simulink model "bpsk_rx_time_sync"  (R2019a)
settings: Solver=VariableStepAuto  StartTime=0.0  StopTime=4000/3.2e6  RelTol=1e-3
InitFcn:
  | setup_bpsk_receiver
undefined symbols (not defined in the file): AXI4, designMultirateFIR, Lite, tx_data, xlfda_numerator
libraries: xbsIndex_r4 x34, dspmlti4 x11, hdlsllib x11, dspswit3 x4, dspsigops x2, commrandsrc3 x1, simulink x1
(part 1 of 2)
settings Model: Creator=david  LastModifiedBy=david

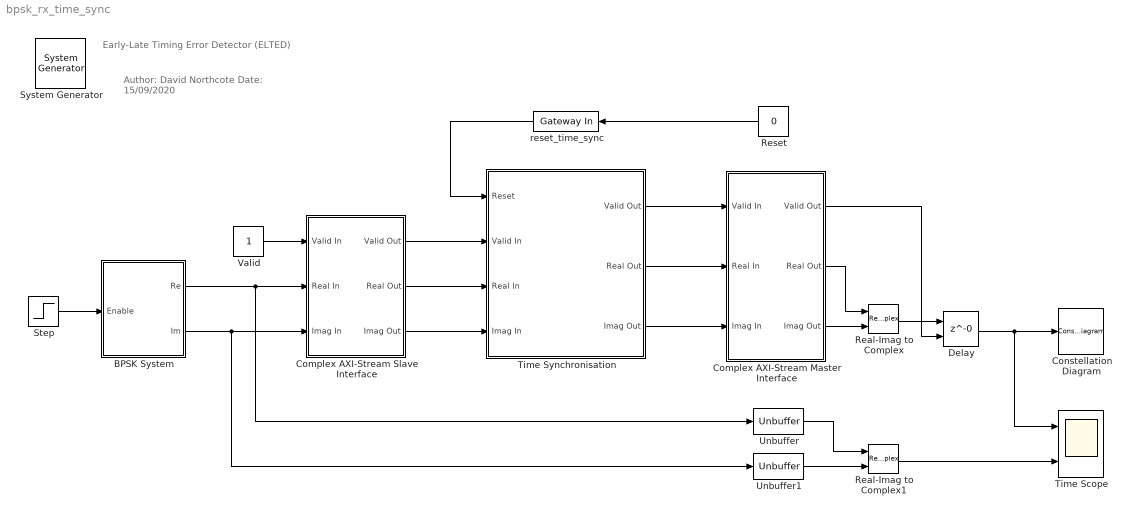
== system bpsk_rx_time_sync ==
  note: Author: 	David Northcote
      | Date: 	15/09/2020
  note: Early-Late Timing Error Detector (ELTED)
  " System Generator" : xbsIndex_r4/ System Generator  Tag=genX  xilinxfamily=zynquplusRFSOC  part=xczu28dr  speed=-2-e  package=ffvg1517  synthesis_tool=Vivado  clock_wrapper=Clock Enables  directory=./netlist  proj_type=Vivado  Synth_file=Vivado Synthesis Defaults  Impl_file=Vivado Implementation Defaults  testbench=off  simulink_period=1/3.2e6  sysclk_period=(1/3.2e6)*1e9  dcm_input_clock_period=10  incr_netlist=off  trim_vbits=Everywhere in SubSystem  dbl_ovrd=According to Block Masks  core_generation=According to Block Masks  run_coregen=off  deprecated_control=off  eval_field=0  block_type=sysgen
  BPSK System : Subsystem
  Complex AXI-Stream Master Interface : Subsystem
  Complex AXI-Stream Slave Interface : Subsystem
  Constellation Diagram : ConstellationDiagram
  Delay : Delay  DelayLength=0  ShowEnablePort=on
      settings: InputPortMap=u0,e6
  Real-Imag to Complex : RealImagToComplex
  Real-Imag to Complex1 : RealImagToComplex
  Reset : Constant  Value=0  OutDataTypeStr=boolean  SampleTime=-1
  Step : Step  Time=4/12.5e3  SampleTime=1/12.5e3
  Time Scope : Scope  NumInputPorts=2
  Time Synchronisation : Subsystem
  Unbuffer : Unbuffer
  Unbuffer1 : Unbuffer
  Valid : Constant  OutDataTypeStr=boolean  SampleTime=1/3.2e6
  reset_time_sync : xbsIndex_r4/Gateway In  gui_display_data_type=Boolean  arith_type=Boolean  n_bits=16  bin_pt=14  preci_type=Single  exp_width=8  frac_width=24  rows=1  columns=1  quantization="Round  (unbiased: +/- Inf)"  overflow=Saturate  period=1/3.2e6  UseAsADC=off  ADCChannel='1'  interface=AXI4-Lite  automatic_assignment=off  address_offset=0  intf_name=''  intf_description=''  default_value=0  timing_constraint=None  locs_specified=off  LOCs={}  io_standard={}  inherit_from_input=off  hdl_port=on  dbl_ovrd=off  block_type=gatewayin
  wires:
  BPSK System/1(Re) -> Unbuffer/1, Complex AXI-Stream Slave Interface/2(Real In)
  BPSK System/2(Im) -> Unbuffer1/1, Complex AXI-Stream Slave Interface/3(Imag In)
  Step/1 -> BPSK System/1(Enable)
  Unbuffer1/1 -> Real-Imag to Complex1/2
  Unbuffer/1 -> Real-Imag to Complex1/1
  Real-Imag to Complex1/1 -> Time Scope/2
  Time Synchronisation/1(Valid Out) -> Complex AXI-Stream Master Interface/1(Valid In)
  Time Synchronisation/2(Real Out) -> Complex AXI-Stream Master Interface/2(Real In)
  Time Synchronisation/3(Imag Out) -> Complex AXI-Stream Master Interface/3(Imag In)
  Complex AXI-Stream Master Interface/2(Real Out) -> Real-Imag to Complex/1
  Complex AXI-Stream Master Interface/3(Imag Out) -> Real-Imag to Complex/2
  Valid/1 -> Complex AXI-Stream Slave Interface/1(Valid In)
  Complex AXI-Stream Slave Interface/1(Valid Out) -> Time Synchronisation/2(Valid In)
  Complex AXI-Stream Slave Interface/2(Real Out) -> Time Synchronisation/3(Real In)
  Complex AXI-Stream Slave Interface/3(Imag Out) -> Time Synchronisation/4(Imag In)
  reset_time_sync/1 -> Time Synchronisation/1(Reset)
  Reset/1 -> reset_time_sync/1
  Real-Imag to Complex/1 -> Delay/1
  Complex AXI-Stream Master Interface/1(Valid Out) -> Delay/2
  Delay/1 -> Constellation Diagram/1, Time Scope/1

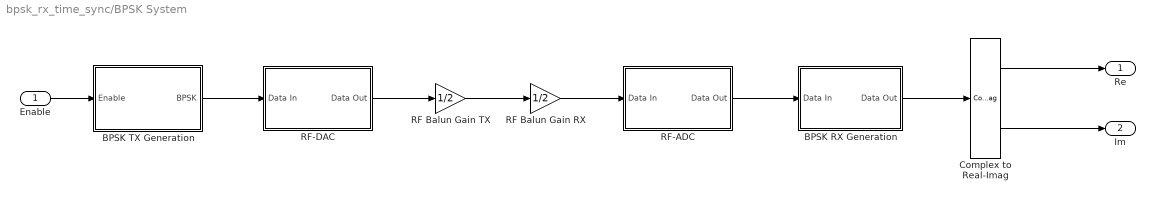
== system bpsk_rx_time_sync/BPSK System ==
  Enable : Inport
  BPSK RX Generation : Subsystem
  BPSK TX Generation : Subsystem
  Complex to Real-Imag : ComplexToRealImag
  RF Balun Gain RX : Gain  Gain=1/2
  RF Balun Gain TX : Gain  Gain=1/2
  RF-ADC : Subsystem  mask{fs_ghz=1.024, decim=8x, ssr=2, mode=Fine, fc=0.064, fph=0, fcoarse=fs/4}
      mask prompts: fs_ghz "Sample Rate (GHz):"; decim "Interpolation Mode:"; ssr "Samples per AXI4-Stream Cycle:"; mode "Mixer Type:"; fc "NCO Frequency (GHz):"; fph "NCO Phase (Rads):"; fcoarse "Frequency:"
      mask init:
      | % Obtain the sample rate in Hz
      | fs = str2double(get_param(gcb, 'fs_ghz'))*1e9;
      | 
      | % Set the mode of the RF-DAC interpolation filter
      | switch get_param(gcb, 'decim')
      |     case '1x'
      |         D = 1;
      |     case '2x'
      |         D = 2;
      |     case '4x'
      |         D = 4;
      |     case '8x'
      |         D = 8;
      |     otherwise
      |         D = 1;
      | end
      | 
      | % Get the AXI-Stream clock for display to user
      | axi_clk = (fs/(str2double(get_param(gcb, 'ssr'))*D))*1e-6;
      | 
      | % Get the block mask object to manipulate settings
      | mo = get_param(gcb, 'MaskObject');
      | 
      | % Update text to display the required AXI-Stream clock
      | tc = mo.getDialogControl('axi_text');
      | tc.Prompt = ['      Required AXI-Stream Clock: ', num2str(axi_clk), ' MHz'];
      | 
      | % Set the RF-DAC Mixer mode
      | switch get_param(gcb, 'mode')
      |     case 'Bypass'
      |         m = 0;
      |     case 'Coarse'
      |         m = 1;
      |     case 'Fine'
      |         m = 2;
      |     otherwise
      |         m = 0;
      | end
      | 
      | % Set the RF-DAC Coarse Mixer mode
      | switch get_param(gcb, 'fcoarse')
      |     case 'fs/2'
      |         mc = 0;
      |     case 'fs/4'
      |         mc = 1;
      |     case '-fs/4'
      |         mc = 2;
      |     otherwise
      |         mc = 0;
      | end
      | 
      | % Set other blocks
      | set_param([gcb, '/Decimation Filter'], 'decim', get_param(gcb, 'decim'));
      mask Callback fs_ghz:
      | % Obtain the sample rate in Hz
      | fs = str2double(get_param(gcb, 'fs_ghz'))*1e9;
      | 
      | % Set the mode of the RF-DAC interpolation filter
      | switch get_param(gcb, 'decim')
      |     case '1x'
      |         D = 1;
      |     case '2x'
      |         D = 2;
      |     case '4x'
      |         D = 4;
      |     case '8x'
      |         D = 8;
      |     otherwise
      |         D = 1;
      | end
      | 
      | % Get the AXI-Stream clock for display to user
      | axi_clk = (fs/(str2double(get_param(gcb, 'ssr'))*D))*1e-6;
      | 
      | % Get the block mask object to manipulate settings
      | mo = get_param(gcb, 'MaskObject');
      | 
      | % Update text to display the required AXI-Stream clock
      | tc = mo.getDialogControl('axi_text');
      | tc.Prompt = ['      Required AXI-Stream Clock: ', num2str(axi_clk), ' MHz'];
      mask TypeOptions decim: 1x | 2x | 4x | 8x
      mask Callback decim:
      | % Obtain the sample rate in Hz
      | fs = str2double(get_param(gcb, 'fs_ghz'))*1e9;
      | 
      | % Set the mode of the RF-DAC interpolation filter
      | switch get_param(gcb, 'decim')
      |     case '1x'
      |         D = 1;
      |     case '2x'
      |         D = 2;
      |     case '4x'
      |         D = 4;
      |     case '8x'
      |         D = 8;
      |     otherwise
      |         D = 1;
      | end
      | 
      | % Get the AXI-Stream clock for display to user
      | axi_clk = (fs/(str2double(get_param(gcb, 'ssr'))*D))*1e-6;
      | 
      | % Get the block mask object to manipulate settings
      | mo = get_param(gcb, 'MaskObject');
      | 
      | % Update text to display the required AXI-Stream clock
      | tc = mo.getDialogControl('axi_text');
      | tc.Prompt = ['      Required AXI-Stream Clock: ', num2str(axi_clk), ' MHz'];
      mask TypeOptions ssr: 1 | 2 | 3 | 4 | 5 | 6 | 7 | 8 | 9 | 10 | 11 | 12 | 13 | 14 | 15 | 16
      mask Callback ssr:
      | % Obtain the sample rate in Hz
      | fs = str2double(get_param(gcb, 'fs_ghz'))*1e9;
      | 
      | % Set the mode of the RF-DAC interpolation filter
      | switch get_param(gcb, 'decim')
      |     case '1x'
      |         D = 1;
      |     case '2x'
      |         D = 2;
      |     case '4x'
      |         D = 4;
      |     case '8x'
      |         D = 8;
      |     otherwise
      |         D = 1;
      | end
      | 
      | % Get the AXI-Stream clock for display to user
      | axi_clk = (fs/(str2double(get_param(gcb, 'ssr'))*D))*1e-6;
      | 
      | % Get the block mask object to manipulate settings
      | mo = get_param(gcb, 'MaskObject');
      | 
      | % Update text to display the required AXI-Stream clock
      | tc = mo.getDialogControl('axi_text');
      | tc.Prompt = ['      Required AXI-Stream Clock: ', num2str(axi_clk), ' MHz'];
      mask TypeOptions mode: Coarse | Fine
      mask Callback mode:
      | % Get the block mask object to manipulate settings
      | mo = get_param(gcb, 'MaskObject');
      | 
      | % Hide group depending on Mixer mode choice
      | switch get_param(gcb, 'mode')
      |     case 'Bypass'
      |         mo.getDialogControl('coarse_group').Visible='off';
      |         mo.getDialogControl('mixer_group').Visible='off';
      |     case 'Coarse'
      |         mo.getDialogControl('coarse_group').Visible='on';
      |         mo.getDialogControl('mixer_group').Visible='off';
      |     case 'Fine'
      |         mo.getDialogControl('coarse_group').Visible='off';
      |         mo.getDialogControl('mixer_group').Visible='on';
      |     otherwise
      |         mo.getDialogControl('coarse_group').Visible='off';
      |         mo.getDialogControl('mixer_group').Visible='off';
      | end
      mask TypeOptions fcoarse: fs/2 | fs/4 | -fs/4
      mask DialogControl DescGroupVar Prompt: RF-DAC
      mask DialogControl DescTextVar Prompt: This block simulates one RF-ADC channel.
      mask DialogControl main_group Prompt: Data Settings
      mask DialogControl axi_text Prompt: Required AXI-Stream Clock: 64 MHz
      mask DialogControl Container5 Prompt: Mixer Settings
  RF-DAC : Subsystem  mask{fs_ghz=1.024, interp=8x, ssr=1, mode=Fine, fc=0.064, fph=0, fcoarse=fs/4}
      mask prompts: fs_ghz "Sample Rate (GHz):"; interp "Interpolation Mode:"; ssr "Samples per AXI4-Stream Cycle:"; mode "Mixer Type:"; fc "NCO Frequency (GHz):"; fph "NCO Phase (Rads):"; fcoarse "Frequency:"
      mask init:
      | % Obtain the sample rate in Hz
      | fs = str2double(get_param(gcb, 'fs_ghz'))*1e9;
      | 
      | % Set the mode of the RF-DAC interpolation filter
      | switch get_param(gcb, 'interp')
      |     case '1x'
      |         L = 1;
      |     case '2x'
      |         L = 2;
      |     case '4x'
      |         L = 4;
      |     case '8x'
      |         L = 8;
      |     otherwise
      |         L = 1;
      | end
      | 
      | % Get the AXI-Stream clock for display to user
      | axi_clk = (fs/(str2double(get_param(gcb, 'ssr'))*L))*1e-6;
      | 
      | % Get the block mask object to manipulate settings
      | mo = get_param(gcb, 'MaskObject');
      | 
      | % Update text to display the required AXI-Stream clock
      | tc = mo.getDialogControl('axi_text');
      | tc.Prompt = ['      Required AXI-Stream Clock: ', num2str(axi_clk), ' MHz'];
      | 
      | % Set the RF-DAC Mixer mode
      | switch get_param(gcb, 'mode')
      |     case 'Bypass'
      |         m = 0;
      |     case 'Coarse'
      |         m = 1;
      |     case 'Fine'
      |         m = 2;
      |     otherwise
      |         m = 0;
      | end
      | 
      | % Set the RF-DAC Coarse Mixer mode
      | switch get_param(gcb, 'fcoarse')
      |     case 'fs/2'
      |         mc = 0;
      |     case 'fs/4'
      |         mc = 1;
      |     case '-fs/4'
      |         mc = 2;
      |     otherwise
      |         mc = 0;
      | end
      | 
      | % Set other blocks
      | set_param([gcb, '/Interpolation Filter'], 'interp', get_param(gcb, 'interp'));
      mask Callback fs_ghz:
      | % Obtain the sample rate in Hz
      | fs = str2double(get_param(gcb, 'fs_ghz'))*1e9;
      | 
      | % Set the mode of the RF-DAC interpolation filter
      | switch get_param(gcb, 'interp')
      |     case '1x'
      |         L = 1;
      |     case '2x'
      |         L = 2;
      |     case '4x'
      |         L = 4;
      |     case '8x'
      |         L = 8;
      |     otherwise
      |         L = 1;
      | end
      | 
      | % Get the AXI-Stream clock for display to user
      | axi_clk = (fs/(str2double(get_param(gcb, 'ssr'))*L))*1e-6;
      | 
      | % Get the block mask object to manipulate settings
      | mo = get_param(gcb, 'MaskObject');
      | 
      | % Update text to display the required AXI-Stream clock
      | tc = mo.getDialogControl('axi_text');
      | tc.Prompt = ['      Required AXI-Stream Clock: ', num2str(axi_clk), ' MHz'];
      mask TypeOptions interp: 1x | 2x | 4x | 8x
      mask Callback interp:
      | % Obtain the sample rate in Hz
      | fs = str2double(get_param(gcb, 'fs_ghz'))*1e9;
      | 
      | % Set the mode of the RF-DAC interpolation filter
      | switch get_param(gcb, 'interp')
      |     case '1x'
      |         L = 1;
      |     case '2x'
      |         L = 2;
      |     case '4x'
      |         L = 4;
      |     case '8x'
      |         L = 8;
      |     otherwise
      |         L = 1;
      | end
      | 
      | % Get the AXI-Stream clock for display to user
      | axi_clk = (fs/(str2double(get_param(gcb, 'ssr'))*L))*1e-6;
      | 
      | % Get the block mask object to manipulate settings
      | mo = get_param(gcb, 'MaskObject');
      | 
      | % Update text to display the required AXI-Stream clock
      | tc = mo.getDialogControl('axi_text');
      | tc.Prompt = ['      Required AXI-Stream Clock: ', num2str(axi_clk), ' MHz'];
      mask TypeOptions ssr: 1 | 2 | 3 | 4 | 5 | 6 | 7 | 8 | 9 | 10 | 11 | 12 | 13 | 14 | 15 | 16
      mask Callback ssr:
      | % Obtain the sample rate in Hz
      | fs = str2double(get_param(gcb, 'fs_ghz'))*1e9;
      | 
      | % Set the mode of the RF-DAC interpolation filter
      | switch get_param(gcb, 'interp')
      |     case '1x'
      |         L = 1;
      |     case '2x'
      |         L = 2;
      |     case '4x'
      |         L = 4;
      |     case '8x'
      |         L = 8;
      |     otherwise
      |         L = 1;
      | end
      | 
      | % Get the AXI-Stream clock for display to user
      | axi_clk = (fs/(str2double(get_param(gcb, 'ssr'))*L))*1e-6;
      | 
      | % Get the block mask object to manipulate settings
      | mo = get_param(gcb, 'MaskObject');
      | 
      | % Update text to display the required AXI-Stream clock
      | tc = mo.getDialogControl('axi_text');
      | tc.Prompt = ['      Required AXI-Stream Clock: ', num2str(axi_clk), ' MHz'];
      mask TypeOptions mode: Coarse | Fine
      mask Callback mode:
      | % Get the block mask object to manipulate settings
      | mo = get_param(gcb, 'MaskObject');
      | 
      | % Hide group depending on Mixer mode choice
      | switch get_param(gcb, 'mode')
      |     case 'Bypass'
      |         mo.getDialogControl('coarse_group').Visible='off';
      |         mo.getDialogControl('mixer_group').Visible='off';
      |     case 'Coarse'
      |         mo.getDialogControl('coarse_group').Visible='on';
      |         mo.getDialogControl('mixer_group').Visible='off';
      |     case 'Fine'
      |         mo.getDialogControl('coarse_group').Visible='off';
      |         mo.getDialogControl('mixer_group').Visible='on';
      |     otherwise
      |         mo.getDialogControl('coarse_group').Visible='off';
      |         mo.getDialogControl('mixer_group').Visible='off';
      | end
      mask TypeOptions fcoarse: fs/2 | fs/4 | -fs/4
      mask DialogControl DescGroupVar Prompt: RF-DAC
      mask DialogControl DescTextVar Prompt: This block simulates one RF-DAC channel.
      mask DialogControl main_group Prompt: Data Settings
      mask DialogControl axi_text Prompt: Required AXI-Stream Clock: 128 MHz
      mask DialogControl Container5 Prompt: Mixer Settings
  Re : Outport
  Im : Outport  Port=2
  wires:
  RF Balun Gain RX/1 -> RF-ADC/1(Data In)
  RF Balun Gain TX/1 -> RF Balun Gain RX/1
  RF-DAC/1(Data Out) -> RF Balun Gain TX/1
  Complex to Real-Imag/2 -> Im/1
  Complex to Real-Imag/1 -> Re/1
  Enable/1 -> BPSK TX Generation/1(Enable)
  BPSK TX Generation/1(BPSK) -> RF-DAC/1(Data In)
  RF-ADC/1(Data Out) -> BPSK RX Generation/1(Data In)
  BPSK RX Generation/1(Data Out) -> Complex to Real-Imag/1

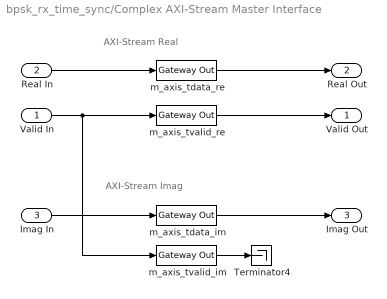
== system bpsk_rx_time_sync/Complex AXI-Stream Master Interface ==
  note: AXI-Stream Real
  note: AXI-Stream Imag
  Valid In : Inport
  Real In : Inport  Port=2
  Imag In : Inport  Port=3
  Terminator4 : Terminator
  m_axis_tdata_im : xbsIndex_r4/Gateway Out  inherit_from_input=off  hdl_port=on  rows=1  columns=1  UseAsDAC=off  DACChannel='1'  interface=None  automatic_assignment=on  address_offset=hex2dec('00')  intf_name=''  intf_description=''  timing_constraint=None  locs_specified=off  LOCs={}  io_standard={}  block_type=gatewayout
  m_axis_tdata_re : xbsIndex_r4/Gateway Out  inherit_from_input=off  hdl_port=on  rows=1  columns=1  UseAsDAC=off  DACChannel='1'  interface=None  automatic_assignment=on  address_offset=hex2dec('00')  intf_name=''  intf_description=''  timing_constraint=None  locs_specified=off  LOCs={}  io_standard={}  block_type=gatewayout
  m_axis_tvalid_im : xbsIndex_r4/Gateway Out  inherit_from_input=off  hdl_port=on  rows=1  columns=1  UseAsDAC=off  DACChannel='1'  interface=None  automatic_assignment=on  address_offset=hex2dec('00')  intf_name=''  intf_description=''  timing_constraint=None  locs_specified=off  LOCs={}  io_standard={}  block_type=gatewayout
  m_axis_tvalid_re : xbsIndex_r4/Gateway Out  inherit_from_input=off  hdl_port=on  rows=1  columns=1  UseAsDAC=off  DACChannel='1'  interface=None  automatic_assignment=on  address_offset=hex2dec('00')  intf_name=''  intf_description=''  timing_constraint=None  locs_specified=off  LOCs={}  io_standard={}  block_type=gatewayout
  Valid Out : Outport
  Real Out : Outport  Port=2
  Imag Out : Outport  Port=3
  wires:
  Real In/1 -> m_axis_tdata_re/1
  m_axis_tdata_im/1 -> Imag Out/1
  m_axis_tvalid_im/1 -> Terminator4/1
  Valid In/1 -> m_axis_tvalid_re/1, m_axis_tvalid_im/1
  m_axis_tdata_re/1 -> Real Out/1
  m_axis_tvalid_re/1 -> Valid Out/1
  Imag In/1 -> m_axis_tdata_im/1

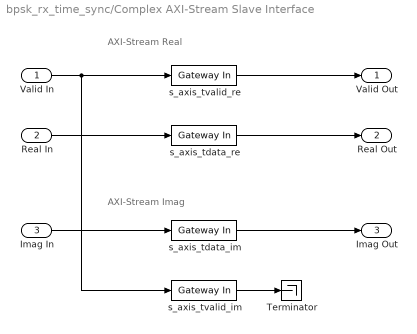
== system bpsk_rx_time_sync/Complex AXI-Stream Slave Interface ==
  note: AXI-Stream Real
  note: AXI-Stream Imag
  Valid In : Inport
  Real In : Inport  Port=2
  Imag In : Inport  Port=3
  Terminator : Terminator
  s_axis_tdata_im : xbsIndex_r4/Gateway In  gui_display_data_type=Fixed-point  arith_type="Signed  (2's comp)"  n_bits=16  bin_pt=14  preci_type=Single  exp_width=8  frac_width=24  rows=1  columns=1  quantization="Round  (unbiased: +/- Inf)"  overflow=Saturate  period=1/3.2e6  UseAsADC=off  ADCChannel='1'  interface=None  automatic_assignment=on  address_offset=hex2dec('00')  intf_name=''  intf_description=''  default_value=0  timing_constraint=None  locs_specified=off  LOCs={}  io_standard={}  inherit_from_input=off  hdl_port=on  dbl_ovrd=off  block_type=gatewayin
  s_axis_tdata_re : xbsIndex_r4/Gateway In  gui_display_data_type=Fixed-point  arith_type="Signed  (2's comp)"  n_bits=16  bin_pt=14  preci_type=Single  exp_width=8  frac_width=24  rows=1  columns=1  quantization="Round  (unbiased: +/- Inf)"  overflow=Saturate  period=1/3.2e6  UseAsADC=off  ADCChannel='1'  interface=None  automatic_assignment=on  address_offset=hex2dec('00')  intf_name=''  intf_description=''  default_value=0  timing_constraint=None  locs_specified=off  LOCs={}  io_standard={}  inherit_from_input=off  hdl_port=on  dbl_ovrd=off  block_type=gatewayin
  s_axis_tvalid_im : xbsIndex_r4/Gateway In  gui_display_data_type=Boolean  arith_type=Boolean  n_bits=16  bin_pt=14  preci_type=Single  exp_width=8  frac_width=24  rows=1  columns=1  quantization="Round  (unbiased: +/- Inf)"  overflow=Saturate  period=1/3.2e6  UseAsADC=off  ADCChannel='1'  interface=None  automatic_assignment=on  address_offset=hex2dec('00')  intf_name=''  intf_description=''  default_value=0  timing_constraint=None  locs_specified=off  LOCs={}  io_standard={}  inherit_from_input=off  hdl_port=on  dbl_ovrd=off  block_type=gatewayin
  s_axis_tvalid_re : xbsIndex_r4/Gateway In  gui_display_data_type=Boolean  arith_type=Boolean  n_bits=16  bin_pt=14  preci_type=Single  exp_width=8  frac_width=24  rows=1  columns=1  quantization="Round  (unbiased: +/- Inf)"  overflow=Saturate  period=1/3.2e6  UseAsADC=off  ADCChannel='1'  interface=None  automatic_assignment=on  address_offset=hex2dec('00')  intf_name=''  intf_description=''  default_value=0  timing_constraint=None  locs_specified=off  LOCs={}  io_standard={}  inherit_from_input=off  hdl_port=on  dbl_ovrd=off  block_type=gatewayin
  Valid Out : Outport
  Real Out : Outport  Port=2
  Imag Out : Outport  Port=3
  wires:
  Imag In/1 -> s_axis_tdata_im/1
  s_axis_tdata_re/1 -> Real Out/1
  s_axis_tdata_im/1 -> Imag Out/1
  Valid In/1 -> s_axis_tvalid_im/1, s_axis_tvalid_re/1
  s_axis_tvalid_re/1 -> Valid Out/1
  s_axis_tvalid_im/1 -> Terminator/1
  Real In/1 -> s_axis_tdata_re/1

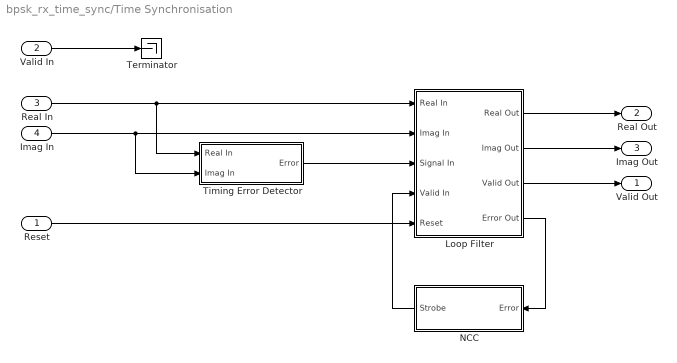
== system bpsk_rx_time_sync/Time Synchronisation ==
  Reset : Inport
  Valid In : Inport  Port=2
  Real In : Inport  Port=3
  Imag In : Inport  Port=4
  Loop Filter : Subsystem  mask{T=1/100e3, d=1/sqrt(2), Kp=3.7, Bn=0.01*100e3, Ko=1}
      mask prompts: T "Sampling Period:"; d "Damping Ratio:"; Kp "Phase Detector Gain:"; Bn "Noise Bandwidth:"; Ko "Oscillator Gain:"
      mask init:
      | n = (Bn*T)/(d+1/(4*d));
      | 
      | K1 = ((4*d*n)/(1+2*d*n+n^2))/(Ko*Kp);
      | 
      | K2 = ((4*n^2)/(1+2*d*n+n^2))/(Ko*Kp);
      | 
      | %K1 = (4*d*n)/(Ko*Kp);
      | 
      | %K2 = (4*(n^2))/(Ko*Kp);
      mask DialogControl DescGroupVar Prompt: Loop Filter
      mask DialogControl DescTextVar Prompt: A simplified loop filter.
      mask DialogControl ParameterGroupVar Prompt: Main
  NCC : Subsystem  mask{r=32}
      mask prompts: r "Symbol Oversample Factor:"
      mask init:
      | n = ceil(log2(r));
      | f = 32-n;
      mask DialogControl DescGroupVar Prompt: Numerically Controlled Clock (NCC)
      mask DialogControl DescTextVar Prompt: The NCC block contains an accumulator that increments by one each clock cycle. The wordlength of the accumulator is determined by the symbol oversampling factor. Once the maximum value of the accumulator is reached, the accumulation starts again. The error signal can be used to increase or decrease the rate of accumulation. When the accumulator wraps around, a binary high is released from the strobe port.
      mask DialogControl ParameterGroupVar Prompt: Main
  Terminator : Terminator
  Timing Error Detector : Subsystem
  Valid Out : Outport
  Real Out : Outport  Port=2
  Imag Out : Outport  Port=3
  wires:
  Reset/1 -> Loop Filter/5(Reset)
  NCC/1(Strobe) -> Loop Filter/4(Valid In)
  Loop Filter/2(Imag Out) -> Imag Out/1
  Loop Filter/1(Real Out) -> Real Out/1
  Loop Filter/3(Valid Out) -> Valid Out/1
  Imag In/1 -> Timing Error Detector/2(Imag In), Loop Filter/2(Imag In)
  Timing Error Detector/1(Error) -> Loop Filter/3(Signal In)
  Loop Filter/4(Error Out) -> NCC/1(Error)
  Real In/1 -> Loop Filter/1(Real In), Timing Error Detector/1(Real In)
  Valid In/1 -> Terminator/1

== system bpsk_rx_time_sync/BPSK System/BPSK RX Generation ==
  Data In : Inport
  CIC Decimation : dspmlti4/CIC Decimation  filtFrom=Dialog parameters  filtobj=CICDECIM  ftype=Decimator  R=5  M=1  N=3  filterInternals=Full precision  BPS=[16 16 16 16]  FLPS=0  outputWordLength=32  outputFracLength=0  launchFVT=off  framing=Maintain input frame rate  RateOptions=Allow multirate processing
      settings: SourceProductName=DSP System Toolbox  SourceProductBaseCode=DS
  FDATool : xbsIndex_r4/FDATool  block_type=fdatool
      settings: infoedit=FDATool
  FIR 0 : dspmlti4/FIR Decimation  FilterSource=Dialog parameters  h=xlfda_numerator('FDATool')/(max(xlfda_numerator('FDATool'))*2)  D=2  filtStruct=Direct form  FilterObject=fir0  framing=Enforce single-rate processing  inputOffset=0  outputBufInitCond=0  roundingMode=Floor  overflowMode=off  firstCoeffDataTypeStr=Inherit: Same word length as input  firstCoeffMin=[]  firstCoeffMax=[]  firstCoeffLastDataTypeStr=Inherit: Same word length as input  outputMode=Binary point scaling  outputWordLength=16  outputFracLength=14  outputDataTypeStr=fixdt(1,16,14)  outputMin=[]  outputMax=[]  outputLastDataTypeStr=fixdt(1,16,14)
  Gain : Gain  Gain=2^(floor(log2(5^3)))/(5^3)  ParamDataTypeStr=fixdt(1,16,14)  OutDataTypeStr=fixdt(1,16,14)
  RRC Receive Filter : Subsystem
  Shift Arithmetic : ArithShift  BitShiftNumber=floor(log2(5^3))  BitShiftDirection=Right
  Unbuffer : Unbuffer
  Data Out : Outport
  wires:
  Unbuffer/1 -> FIR 0/1
  Data In/1 -> Unbuffer/1
  FIR 0/1 -> CIC Decimation/1
  CIC Decimation/1 -> Shift Arithmetic/1
  Shift Arithmetic/1 -> Gain/1
  Gain/1 -> RRC Receive Filter/1(Data In)
  RRC Receive Filter/1(Data Out) -> Data Out/1

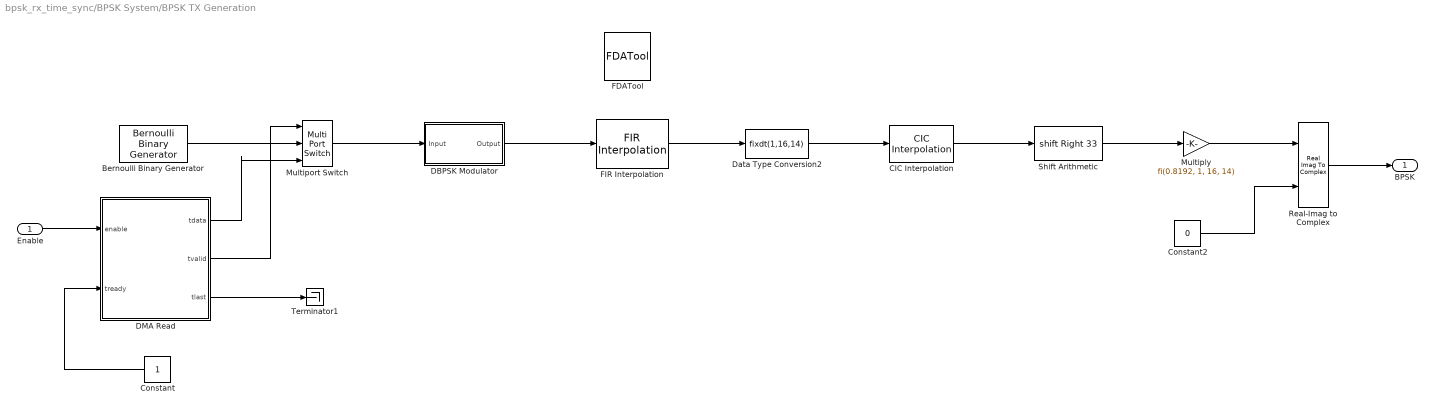
== system bpsk_rx_time_sync/BPSK System/BPSK TX Generation ==
  Enable : Inport
  Bernoulli Binary Generator : commrandsrc3/Bernoulli Binary Generator  ProbabilityOfZero=0.5  SeedSource=Auto  Seed=0  SampleTime=1/100e3  SamplesPerFrame=1  OutputDataType=double  SimulateUsing=Interpreted execution
      settings: SourceProductName=Communications Toolbox
  CIC Interpolation : dspmlti4/CIC Interpolation  filtFrom=Dialog parameters  filtobj=Hm_interp  ftype=Interpolator  R=320  M=1  N=5  filterInternals=Full precision  BPS=[16 16 16 16]  FLPS=0  outputWordLength=32  outputFracLength=0  launchFVT=off  framing=Allow multirate processing  OutputFrames=off
      settings: SourceProductName=DSP System Toolbox  SourceProductBaseCode=DS
  Constant : Constant  SampleTime=1/12.5e3
  Constant2 : Constant  Value=0  OutDataTypeStr=Inherit: Inherit via back propagation  SampleTime=-1
  DBPSK Modulator : Subsystem
  DMA Read : Subsystem
  Data Type Conversion2 : DataTypeConversion  OutDataTypeStr=fixdt(1,16,14)
  FDATool : xbsIndex_r4/FDATool  block_type=fdatool
      settings: infoedit=FDATool
  FIR Interpolation : dspmlti4/FIR Interpolation  FilterSource=Dialog parameters  h=xlfda_numerator('FDATool')/(max(xlfda_numerator('FDATool')))  L=4  FilterObject=xlfda_numerator('FDATool')/(max(xlfda_numerator('FDATool')))  framing=Allow multirate processing  outputBufInitCond=0  roundingMode=Floor  overflowMode=off  firstCoeffMode=Binary point scaling  firstCoeffWordLength=16  firstCoeffFracLength=14  firstCoeffDataTypeStr=fixdt(1,16,14)  firstCoeffMin=[]  firstCoeffMax=[]  firstCoeffLastDataTypeStr=fixdt(1,16,14)  outputDataTypeStr=Inherit: Same as accumulator  outputMin=[]  outputMax=[]  outputLastDataTypeStr=Inherit: Same as accumulator
      settings: SourceProductName=DSP System Toolbox
  Multiply : Gain  Gain=fi(0.8192, 1, 16, 14)  ParamDataTypeStr=fixdt(1,16,15)  OutDataTypeStr=fixdt(1,16,14)
  Multiport Switch : MultiPortSwitch  DataPortOrder=Zero-based contiguous  Inputs=2  zeroidx=on
  Real-Imag to Complex : RealImagToComplex
  Shift Arithmetic : ArithShift  BitShiftNumber=33  BitShiftDirection=Right
  Terminator1 : Terminator
  BPSK : Outport
  wires:
  Shift Arithmetic/1 -> Multiply/1
  Data Type Conversion2/1 -> CIC Interpolation/1
  DBPSK Modulator/1(Output) -> FIR Interpolation/1
  Multiport Switch/1 -> DBPSK Modulator/1(Input)
  Constant/1 -> DMA Read/2(tready)
  Enable/1 -> DMA Read/1(enable)
  DMA Read/3(tlast) -> Terminator1/1
  DMA Read/1(tdata) -> Multiport Switch/3
  DMA Read/2(tvalid) -> Multiport Switch/1
  Bernoulli Binary Generator/1 -> Multiport Switch/2
  FIR Interpolation/1 -> Data Type Conversion2/1
  CIC Interpolation/1 -> Shift Arithmetic/1
  Multiply/1 -> Real-Imag to Complex/1
  Real-Imag to Complex/1 -> BPSK/1
  Constant2/1 -> Real-Imag to Complex/2

== system bpsk_rx_time_sync/BPSK System/RF-ADC ==
  Data In : Inport
  Decimation Filter : Subsystem  mask{decim=8x}
      mask prompts: decim "Decimation Factor:"
      mask init:
      | fir0 = dsp.FIRDecimator('DecimationFactor', 2,...
      |                            'CoefficientsDataType', 'Custom',...
      |                            'CustomCoefficientsDataType', numerictype([], 16, 14),...
      |                            'FullPrecisionOverride', false,...
      |                            'OutputDataType', 'Custom',...
      |                            'CustomOutputDataType', numerictype([], 16, 14),...
      |                            'Numerator', [-6, 0 54, 0, -254, 0, 1230, 2048, 1230, 0, -254, 0, 54, 0, -6]/(2048*2));
      | fir1 = dsp.FIRDecimator('DecimationFactor', 2,...
      |                            'CoefficientsDataType', 'Custom',...
      |                            'CustomCoefficientsDataType', numerictype([], 16, 14),...
      |                            'FullPrecisionOverride', false,...
      |                            'OutputDataType', 'Custom',...
      |                            'CustomOutputDataType', numerictype([], 16, 14),...
      |                            'Numerator', [-12, 0, 84, 0, -337, 0, 1008, 0, -2693, 0, 10142, 16384, 10142, 0, -2693, 0, 1008, 0, -337, 0, 84, 0 ,-12]/(16384*2));
      | fir2 = dsp.FIRDecimator('DecimationFactor', 2,...
      |                            'CoefficientsDataType', 'Custom',...
      |                            'CustomCoefficientsDataType', numerictype([], 16, 14),...
      |                            'FullPrecisionOverride', false,...
      |                            'OutputDataType', 'Custom',...
      |                            'CustomOutputDataType', numerictype([], 16, 14),...
      |                            'Numerator', [5, 0, -17, 0, 44, 0, -96, 0, 187, 0, -335, 0, 565, 0, -906, 0, 1401, 0, -2112, 0, 3145, 0, -4723, 0, 7415, 0, -13331, 0, 41526, 65536, 41526, 0, -13331, 0, 7415, 0, -4723, 0, 3145, 0, -2112, 0, 1401, 0, -906, 0, 565, 0, -335, 0, 187, 0, -96, 0, 44, 0, -17, 0, 5]/(65536));
      | switch get_param(gcb, 'decim')
      |     case '1x'
      |         if ~strcmp(get_param([gcb, '/FIR 0'], 'Commented'), 'through')
      |             set_param([gcb, '/FIR 0'],'Commented','through');
      |         end
      |         
      |         if ~strcmp(get_param([gcb, '/FIR 1'], 'Commented'), 'through')
      |             set_param([gcb, '/FIR 1'],'Commented','through');
      |         end
      |         
      |         if ~strcmp(get_param([gcb, '/FIR 2'], 'Commented'), 'through')
      |             set_param([gcb, '/FIR 2'],'Commented','through');
      |         end
      |             
      |     case '2x'
      |         if ~strcmp(get_param([gcb, '/FIR 0'], 'Commented'), 'through')
      |             set_param([gcb, '/FIR 0'],'Commented','through');
      |         end
      |         
      |         if ~strcmp(get_param([gcb, '/FIR 1'], 'Commented'), 'through')
      |             set_param([gcb, '/FIR 1'],'Commented','through');
      |         end
      |         
      |         if ~strcmp(get_param([gcb, '/FIR 2'], 'Commented'), 'off')
      |             set_param([gcb, '/FIR 2'],'Commented','off');
      |         end
      | 
      |     case '4x'
      |         if ~strcmp(get_param([gcb, '/FIR 0'], 'Commented'), 'through')
      |             set_param([gcb, '/FIR 0'],'Commented','through');
      |         end
      |         
      |         if ~strcmp(get_param([gcb, '/FIR 1'], 'Commented'), 'off')
      |             set_param([gcb, '/FIR 1'],'Commented','off');
      |         end
      |         
      |         if ~strcmp(get_param([gcb, '/FIR 2'], 'Commented'), 'off')
      |             set_param([gcb, '/FIR 2'],'Commented','off');
      |         end
      |         
      |     case '8x'
      |         if ~strcmp(get_param([gcb, '/FIR 0'], 'Commented'), 'off')
      |             set_param([gcb, '/FIR 0'],'Commented','off');
      |         end
      |         
      |         if ~strcmp(get_param([gcb, '/FIR 1'], 'Commented'), 'off')
      |             set_param([gcb, '/FIR 1'],'Commented','off');
      |         end
      |         
      |         if ~strcmp(get_param([gcb, '/FIR 2'], 'Commented'), 'off')
      |             set_param([gcb, '/FIR 2'],'Commented','off');
      |         end
      | 
      | end
      mask TypeOptions decim: 1x | 2x | 4x | 8x
      mask DialogControl DescGroupVar Prompt: RF-DAC Interpolation Filter
      mask DialogControl DescTextVar Prompt: This block simulates the RF-DAC interpolation stage using the same coefficients stored in the interpolation filters.
      mask DialogControl ParameterGroupVar Prompt: Main
  NCO and Mixer : Subsystem
  RF-ADC : Subsystem
  Data Out : Outport
  wires:
  Decimation Filter/1(Data Out) -> Data Out/1
  Data In/1 -> RF-ADC/1(Data In)
  RF-ADC/1(Data Out) -> NCO and Mixer/1(Data In)
  NCO and Mixer/1(Data Out) -> Decimation Filter/1(Data In)

== system bpsk_rx_time_sync/BPSK System/RF-DAC ==
  note: Not Ready
  Data In : Inport
  Coarse Delay : Subsystem
  Interpolation Filter : Subsystem  mask{interp=8x}
      mask prompts: interp "Interpolation Factor:"
      mask init:
      | fir0 = dsp.FIRInterpolator('InterpolationFactor', 2,...
      |                            'CoefficientsDataType', 'Custom',...
      |                            'CustomCoefficientsDataType', numerictype([], 16, 14),...
      |                            'FullPrecisionOverride', false,...
      |                            'OutputDataType', 'Custom',...
      |                            'CustomOutputDataType', numerictype([], 16, 14),...
      |                            'Numerator', [-6, 0 54, 0, -254, 0, 1230, 2048, 1230, 0, -254, 0, 54, 0, -6]/(2048));
      | fir1 = dsp.FIRInterpolator('InterpolationFactor', 2,...
      |                            'CoefficientsDataType', 'Custom',...
      |                            'CustomCoefficientsDataType', numerictype([], 16, 14),...
      |                            'FullPrecisionOverride', false,...
      |                            'OutputDataType', 'Custom',...
      |                            'CustomOutputDataType', numerictype([], 16, 14),...
      |                            'Numerator', [-12, 0, 84, 0, -337, 0, 1008, 0, -2693, 0, 10142, 16384, 10142, 0, -2693, 0, 1008, 0, -337, 0, 84, 0 ,-12]/(16384));
      | fir2 = dsp.FIRInterpolator('InterpolationFactor', 2,...
      |                            'CoefficientsDataType', 'Custom',...
      |                            'CustomCoefficientsDataType', numerictype([], 16, 14),...
      |                            'FullPrecisionOverride', false,...
      |                            'OutputDataType', 'Custom',...
      |                            'CustomOutputDataType', numerictype([], 16, 14),...
      |                            'Numerator', [5, 0, -17, 0, 44, 0, -96, 0, 187, 0, -335, 0, 565, 0, -906, 0, 1401, 0, -2112, 0, 3145, 0, -4723, 0, 7415, 0, -13331, 0, 41526, 65536, 41526, 0, -13331, 0, 7415, 0, -4723, 0, 3145, 0, -2112, 0, 1401, 0, -906, 0, 565, 0, -335, 0, 187, 0, -96, 0, 44, 0, -17, 0, 5]/(65536));
      | switch get_param(gcb, 'interp')
      |     case '1x'
      |         if ~strcmp(get_param([gcb, '/FIR 0'], 'Commented'), 'through')
      |             set_param([gcb, '/FIR 0'],'Commented','through');
      |         end
      |         
      |         if ~strcmp(get_param([gcb, '/FIR 1'], 'Commented'), 'through')
      |             set_param([gcb, '/FIR 1'],'Commented','through');
      |         end
      |         
      |         if ~strcmp(get_param([gcb, '/FIR 2'], 'Commented'), 'through')
      |             set_param([gcb, '/FIR 2'],'Commented','through');
      |         end
      |             
      |     case '2x'
      |         if ~strcmp(get_param([gcb, '/FIR 0'], 'Commented'), 'through')
      |             set_param([gcb, '/FIR 0'],'Commented','through');
      |         end
      |         
      |         if ~strcmp(get_param([gcb, '/FIR 1'], 'Commented'), 'through')
      |             set_param([gcb, '/FIR 1'],'Commented','through');
      |         end
      |         
      |         if ~strcmp(get_param([gcb, '/FIR 2'], 'Commented'), 'off')
      |             set_param([gcb, '/FIR 2'],'Commented','off');
      |         end
      | 
      |     case '4x'
      |         if ~strcmp(get_param([gcb, '/FIR 0'], 'Commented'), 'through')
      |             set_param([gcb, '/FIR 0'],'Commented','through');
      |         end
      |         
      |         if ~strcmp(get_param([gcb, '/FIR 1'], 'Commented'), 'off')
      |             set_param([gcb, '/FIR 1'],'Commented','off');
      |         end
      |         
      |         if ~strcmp(get_param([gcb, '/FIR 2'], 'Commented'), 'off')
      |             set_param([gcb, '/FIR 2'],'Commented','off');
      |         end
      |         
      |     case '8x'
      |         if ~strcmp(get_param([gcb, '/FIR 0'], 'Commented'), 'off')
      |             set_param([gcb, '/FIR 0'],'Commented','off');
      |         end
      |         
      |         if ~strcmp(get_param([gcb, '/FIR 1'], 'Commented'), 'off')
      |             set_param([gcb, '/FIR 1'],'Commented','off');
      |         end
      |         
      |         if ~strcmp(get_param([gcb, '/FIR 2'], 'Commented'), 'off')
      |             set_param([gcb, '/FIR 2'],'Commented','off');
      |         end
      | 
      | end
      mask TypeOptions interp: 1x | 2x | 4x | 8x
      mask DialogControl DescGroupVar Prompt: RF-DAC Interpolation Filter
      mask DialogControl DescTextVar Prompt: This block simulates the RF-DAC interpolation stage using the same coefficients stored in the interpolation filters.
      mask DialogControl ParameterGroupVar Prompt: Main
  NCO and Mixer : Subsystem
  Output Filter : Subsystem
  QMC Gain & Phase : Subsystem
  QMC Threshold : Subsystem
  RF-DAC : Subsystem
  Data Out : Outport
  wires:
  Interpolation Filter/1(Data Out) -> NCO and Mixer/1(Data In)
  NCO and Mixer/1(Data Out) -> QMC Gain & Phase/1(Data In)
  Data In/1 -> Interpolation Filter/1(Data In)
  QMC Gain & Phase/1(Data Out) -> Coarse Delay/1(Data In)
  Coarse Delay/1(Data Out) -> Output Filter/1(Data In)
  Output Filter/1(Data Out) -> QMC Threshold/1(Data In)
  QMC Threshold/1(Data Out) -> RF-DAC/1(Data In)
  RF-DAC/1(Data Out) -> Data Out/1

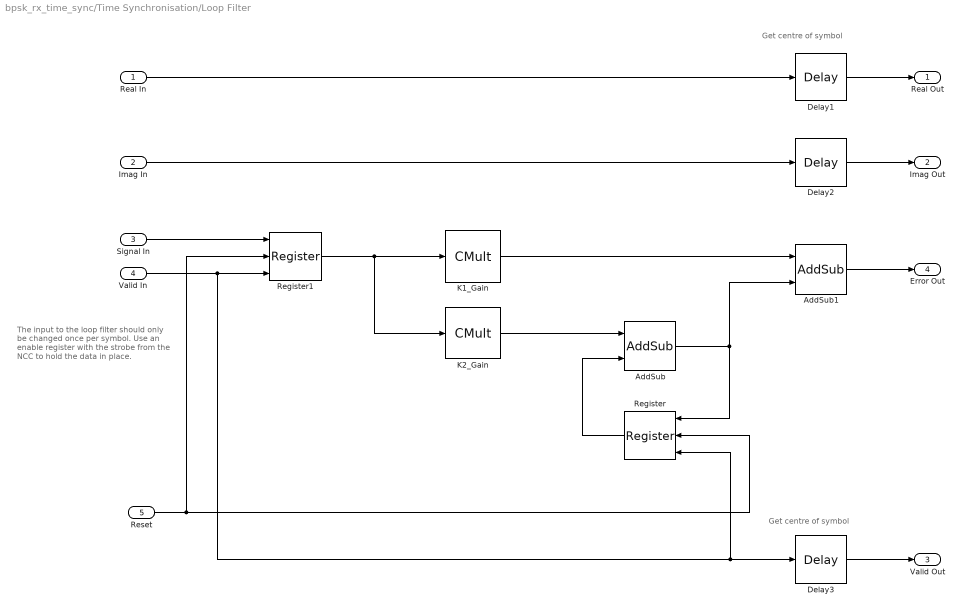
== system bpsk_rx_time_sync/Time Synchronisation/Loop Filter ==
  note: Get centre of symbol
  note: The input to the loop filter should only be changed once per symbol.
      |
      | Use an enable register with the strobe from the NCC to hold the data in place.
  note: Get centre of symbol
  Real In : Inport
  Imag In : Inport  Port=2
  Signal In : Inport  Port=3
  Valid In : Inport  Port=4
  Reset : Inport  Port=5
  AddSub : xbsIndex_r4/AddSub  mode=Addition  use_carryin=off  use_carryout=off  en=off  latency=0  precision=User Defined  arith_type="Signed  (2's comp)"  n_bits=52  bin_pt=44  quantization=Truncate  overflow=Flag as error  use_behavioral_HDL=off  hw_selection=Fabric  pipelined=off  dbl_ovrd=off  block_type=addsub
  AddSub1 : xbsIndex_r4/AddSub  mode=Addition  use_carryin=off  use_carryout=off  en=off  latency=0  precision=Full  arith_type="Signed  (2's comp)"  n_bits=32  bin_pt=31  quantization=Truncate  overflow=Wrap  use_behavioral_HDL=off  hw_selection=Fabric  pipelined=off  dbl_ovrd=off  block_type=addsub
  Delay1 : xbsIndex_r4/Delay  rst=off  infoeditControl=Selection of Reset will increase slice count due to use of real FFs and instead of SRLs  en=off  latency=32/2  reg_retiming=off  dbl_ovrd=off  block_type=delay
  Delay2 : xbsIndex_r4/Delay  rst=off  infoeditControl=Selection of Reset will increase slice count due to use of real FFs and instead of SRLs  en=off  latency=32/2  reg_retiming=off  dbl_ovrd=off  block_type=delay
  Delay3 : xbsIndex_r4/Delay  rst=off  infoeditControl=Selection of Reset will increase slice count due to use of real FFs and instead of SRLs  en=off  latency=32/2  reg_retiming=off  dbl_ovrd=off  block_type=delay
  K1_Gain : xbsIndex_r4/CMult  const=K1  gui_display_data_type=Fixed-point  const_n_bits=18  const_bin_pt=16  float_type=Single  exp_bits=8  fraction_bits=24  en=off  latency=0  precision=Full  arith_type="Signed  (2's comp)"  n_bits=3+28+16  bin_pt=28+16  quantization=Truncate  overflow=Wrap  use_behavioral_HDL=off  mem_type=Distributed RAM  pipeline=off  dbl_ovrd=off  block_type=cmult
  K2_Gain : xbsIndex_r4/CMult  const=K2  gui_display_data_type=Fixed-point  const_n_bits=18  const_bin_pt=16  float_type=Single  exp_bits=8  fraction_bits=24  en=off  latency=0  precision=Full  arith_type="Signed  (2's comp)"  n_bits=3+28+16  bin_pt=28+16  quantization=Truncate  overflow=Wrap  use_behavioral_HDL=off  mem_type=Distributed RAM  pipeline=off  dbl_ovrd=off  block_type=cmult
  Register : xbsIndex_r4/Register  init=0  rst=on  en=on  dbl_ovrd=off  block_type=register
  Register1 : xbsIndex_r4/Register  init=0  rst=on  en=on  dbl_ovrd=off  block_type=register
  Real Out : Outport
  Imag Out : Outport  Port=2
  Valid Out : Outport  Port=3
  Error Out : Outport  Port=4
  wires:
  Delay3/1 -> Valid Out/1
  Reset/1 -> Register/2, Register1/2
  K2_Gain/1 -> AddSub/1
  AddSub1/1 -> Error Out/1
  Real In/1 -> Delay1/1
  Imag In/1 -> Delay2/1
  AddSub/1 -> Register/1, AddSub1/2
  K1_Gain/1 -> AddSub1/1
  Register/1 -> AddSub/2
  Signal In/1 -> Register1/1
  Register1/1 -> K1_Gain/1, K2_Gain/1
  Delay2/1 -> Imag Out/1
  Delay1/1 -> Real Out/1
  Valid In/1 -> Delay3/1, Register/3, Register1/3

== system bpsk_rx_time_sync/Time Synchronisation/NCC ==
  note: For the Numerically Controlled Clock (NCC), we need to consider
      | the symbol oversample factor and the fractional wordlength
      | of the accumulator.
      |
      | The number of samples per symbol determine the maximum value
      | of the accumulator {ceil(log2(n))+1}.
      |
      | The fractional bits determine the quantisation step (precision),
      | of our accumulator.
      |
      | We add 1 to the error signal at all times, as this is necessary to
      | ensure the accumulator always adds 1. If the error is equal to
      | zero, then the accumulator will increase normally. If there is an
      | error in phase not equal to zero, the accumulator will change to
      | compensate for the phase difference.
  Error : Inport
  AddSub : xbsIndex_r4/AddSub  mode=Addition  use_carryin=off  use_carryout=off  en=off  latency=0  precision=User Defined  arith_type=Unsigned  n_bits=n+44  bin_pt=44  quantization=Truncate  overflow=Wrap  use_behavioral_HDL=off  hw_selection=Fabric  pipelined=off  dbl_ovrd=off  block_type=addsub
  AddSub1 : xbsIndex_r4/AddSub  mode=Addition  use_carryin=off  use_carryout=off  en=off  latency=0  precision=Full  arith_type="Signed  (2's comp)"  n_bits=45  bin_pt=44  quantization=Truncate  overflow=Flag as error  use_behavioral_HDL=off  hw_selection=Fabric  pipelined=off  dbl_ovrd=off  block_type=addsub
  Constant : xbsIndex_r4/Constant  const=1  gui_display_data_type=Fixed-point  arith_type=Unsigned  n_bits=1  bin_pt=0  preci_type=Single  exp_width=8  frac_width=24  explicit_period=off  period=1  equ=P=C  opselect=C  inp2=PCIN>>17  opr=+  inp1=P  carry=CIN  dbl_ovrd=off  block_type=constant
  Register : xbsIndex_r4/Register  init=0  rst=off  en=off  dbl_ovrd=off  block_type=register
  Relational : xbsIndex_r4/Relational  mode=a<b  op_type=Bool  en=off  latency=0  dbl_ovrd=off  block_type=relational
  Strobe : Outport
  wires:
  Register/1 -> AddSub/1, Relational/2
  Relational/1 -> Strobe/1
  AddSub/1 -> Register/1, Relational/1
  AddSub1/1 -> AddSub/2
  Constant/1 -> AddSub1/1
  Error/1 -> AddSub1/2

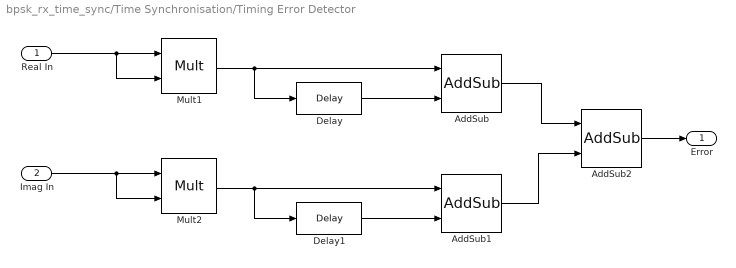
== system bpsk_rx_time_sync/Time Synchronisation/Timing Error Detector ==
  Real In : Inport
  Imag In : Inport  Port=2
  AddSub : xbsIndex_r4/AddSub  mode=Subtraction  use_carryin=off  use_carryout=off  en=off  latency=0  precision=Full  arith_type=Unsigned  n_bits=16  bin_pt=14  quantization=Truncate  overflow=Wrap  use_behavioral_HDL=off  hw_selection=Fabric  pipelined=off  dbl_ovrd=off  block_type=addsub
  AddSub1 : xbsIndex_r4/AddSub  mode=Subtraction  use_carryin=off  use_carryout=off  en=off  latency=0  precision=Full  arith_type=Unsigned  n_bits=16  bin_pt=14  quantization=Truncate  overflow=Wrap  use_behavioral_HDL=off  hw_selection=Fabric  pipelined=off  dbl_ovrd=off  block_type=addsub
  AddSub2 : xbsIndex_r4/AddSub  mode=Addition  use_carryin=off  use_carryout=off  en=off  latency=0  precision=Full  arith_type="Signed  (2's comp)"  n_bits=33  bin_pt=25  quantization="Round  (unbiased: +/- Inf)"  overflow=Saturate  use_behavioral_HDL=off  hw_selection=Fabric  pipelined=off  dbl_ovrd=off  block_type=addsub
  Delay : xbsIndex_r4/Delay  rst=off  infoeditControl=Selection of Reset will increase slice count due to use of real FFs and instead of SRLs  en=off  latency=32  reg_retiming=off  dbl_ovrd=off  block_type=delay
  Delay1 : xbsIndex_r4/Delay  rst=off  infoeditControl=Selection of Reset will increase slice count due to use of real FFs and instead of SRLs  en=off  latency=32  reg_retiming=off  dbl_ovrd=off  block_type=delay
  Mult1 : xbsIndex_r4/Mult  precision=Full  arith_type=Unsigned  n_bits=31  bin_pt=28  quantization=Truncate  overflow=Saturate  en=off  latency=0  use_behavioral_HDL=off  opt=Speed  use_embedded=on  optimum_pipeline=off  pipeline=on  dbl_ovrd=off  use_rpm=on  placement_style=Triangular  block_type=mult
  Mult2 : xbsIndex_r4/Mult  precision=Full  arith_type=Unsigned  n_bits=31  bin_pt=28  quantization=Truncate  overflow=Saturate  en=off  latency=0  use_behavioral_HDL=off  opt=Speed  use_embedded=on  optimum_pipeline=off  pipeline=on  dbl_ovrd=off  use_rpm=on  placement_style=Triangular  block_type=mult
  Error : Outport
  wires:
  Real In/1 -> Mult1/1, Mult1/2
  Imag In/1 -> Mult2/1, Mult2/2
  AddSub/1 -> AddSub2/1
  AddSub2/1 -> Error/1
  Delay1/1 -> AddSub1/2
  Mult2/1 -> Delay1/1, AddSub1/1
  AddSub1/1 -> AddSub2/2
  Mult1/1 -> AddSub/1, Delay/1
  Delay/1 -> AddSub/2

== system bpsk_rx_time_sync/BPSK System/BPSK RX Generation/RRC Receive Filter ==
  Data In : Inport
  Data Type Conversion2 : DataTypeConversion  OutDataTypeStr=fixdt(1,16,14)
  FDATool : xbsIndex_r4/FDATool  block_type=fdatool
      settings: infoedit=FDATool
  FIR Decimation : dspmlti4/FIR Decimation  FilterSource=Dialog parameters  h=xlfda_numerator('FDATool')/(max(xlfda_numerator('FDATool'))*4)  D=4  filtStruct=Direct form  FilterObject=FDECIM  framing=Allow multirate processing  inputOffset=0  outputBufInitCond=0  roundingMode=Floor  overflowMode=off  firstCoeffMode=Binary point scaling  firstCoeffWordLength=16  firstCoeffFracLength=14  firstCoeffDataTypeStr=fixdt(1,16,14)  firstCoeffMin=[]  firstCoeffMax=[]  firstCoeffLastDataTypeStr=fixdt(1,16,14)  outputDataTypeStr=Inherit: Same as accumulator  outputMin=[]  outputMax=[]  outputLastDataTypeStr=Inherit: Same as accumulator
  Data Out : Outport
  wires:
  FIR Decimation/1 -> Data Type Conversion2/1
  Data In/1 -> FIR Decimation/1
  Data Type Conversion2/1 -> Data Out/1

== system bpsk_rx_time_sync/BPSK System/BPSK TX Generation/DBPSK Modulator ==
  Input : Inport
  Cast To Boolean : DataTypeConversion  OutDataTypeStr=boolean
  Constant : Constant  Value=fi(1, 1, 16, 14)  OutDataTypeStr=fixdt(1,16,14)  SampleTime=-1
  Constant1 : Constant  Value=fi(-1, 1, 16, 14)  OutDataTypeStr=fixdt(1,16,14)  SampleTime=-1
  Delay : Delay  DelayLength=1
  Multiport Switch : MultiPortSwitch  DataPortOrder=Zero-based contiguous  Inputs=2  zeroidx=on
  XOR : Logic  Operator=XOR  IconShape=distinctive  AllPortsSameDT=off  OutDataTypeStr=boolean
  Output : Outport
  wires:
  Constant1/1 -> Multiport Switch/3
  Constant/1 -> Multiport Switch/2
  Input/1 -> Cast To Boolean/1
  Delay/1 -> XOR/1
  XOR/1 -> Multiport Switch/1, Delay/1
  Cast To Boolean/1 -> XOR/2
  Multiport Switch/1 -> Output/1
